simulink model "project"  (R2020b)
settings: Solver=VariableStepAuto  StartTime=0.0  StopTime=10  RelTol=1e-3
undefined symbols (not defined in the file or in its folder): sigbuilder_block
settings Model: Creator=99003759  LastModifiedBy=99003759

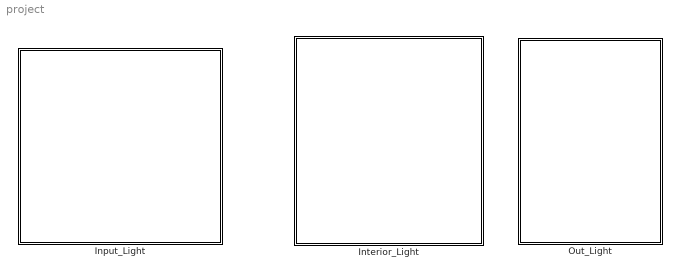
== system project ==
  Input_Light : Subsystem
  Interior_Light : Subsystem
  Out_Light : Subsystem

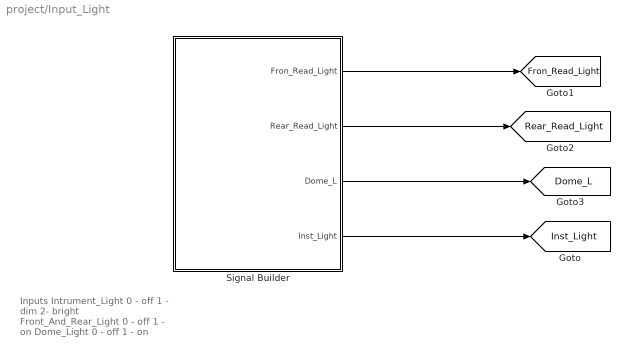
== system project/Input_Light ==
  note: Inputs
      | Intrument_Light
      | 0 - off
      | 1 - dim
      | 2- bright
      | Front_And_Rear_Light
      | 0 - off
      | 1 - on
      | Dome_Light
      | 0 - off
      | 1 - on
  Signal Builder : Subsystem  Tag=STV Subsys  LoadFcn=sigbuilder_block('load');  StartFcn=sigbuilder_block('start');  StopFcn=sigbuilder_block('stop');  ClipboardFcn=sigbuilder_block('clipboard');  mask(Sigbuilder block){tuvar=[0:10]}
      mask help: Simulink:masks:SigbuilderBlock_MD
      mask init:
      | if ~strcmp(get_param(bdroot(gcbh),'SimulationStatus'),'stopped') tuvar = sigbuilder_block('maskInit'); end
      settings: CopyFcn=sigbuilder_block('copy');  DeleteFcn=sigbuilder_block('delete');  ModelCloseFcn=sigbuilder_block('modelClose');  PreSaveFcn=sigbuilder_block('preSave');  PauseFcn=sigbuilder_block('pause');  ContinueFcn=sigbuilder_block('continue');  NameChangeFcn=sigbuilder_block('namechange');  OpenFcn=sigbuilder_block('open',[373.5 207 544.5 355.5 ]);  CloseFcn=sigbuilder_block('close');
      mask Display: plot(0, 0, 100, 100,[2, 2, 32, 32, 2], [68, 8, 8, 68, 68],[32, 2], [38, 38], [32, 19, 2],[53, 60, 44], [32, 17, 17, 2],[16, 16, 31, 31]);txt = getActiveGroup(gcbh);text(2, 100, txt,'verticalAlignment', 'top');
  tag scope: Dome_L=global, Fron_Read_Light=global, Inst_Light=global, Rear_Read_Light=global
  wires:
  Signal Builder/4(Inst_Light) -> [Inst_Light]
  Signal Builder/1(Fron_Read_Light) -> [Fron_Read_Light]
  Signal Builder/2(Rear_Read_Light) -> [Rear_Read_Light]
  Signal Builder/3(Dome_L) -> [Dome_L]

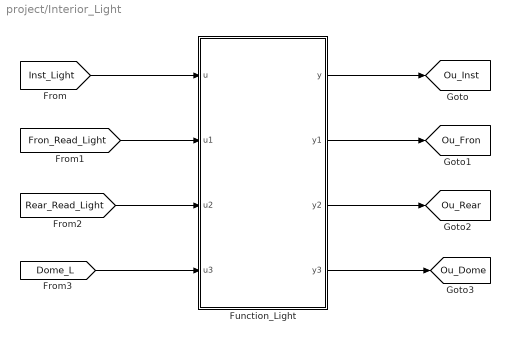
== system project/Interior_Light ==
  Function_Light : MATLAB Function  TreatAsAtomicUnit=on
  tag scope: Ou_Dome=global, Ou_Fron=global, Ou_Inst=global, Ou_Rear=global
  wires:
  [Dome_L] -> Function_Light/4(u3)
  [Inst_Light] -> Function_Light/1(u)
  [Fron_Read_Light] -> Function_Light/2(u1)
  [Rear_Read_Light] -> Function_Light/3(u2)
  Function_Light/1(y) -> [Ou_Inst]
  Function_Light/2(y1) -> [Ou_Fron]
  Function_Light/3(y2) -> [Ou_Rear]
  Function_Light/4(y3) -> [Ou_Dome]

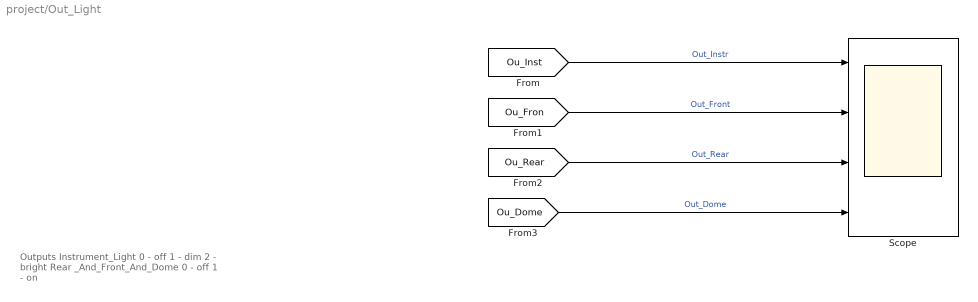
== system project/Out_Light ==
  note: Outputs
      | Instrument_Light
      | 0 - off
      | 1 - dim
      | 2 - bright
      | Rear _And_Front_And_Dome
      | 0 - off
      | 1 - on
  Scope : Scope  NumInputPorts=4
  wires:
  [Ou_Fron] -> Scope/2  "Out_Front"
  [Ou_Rear] -> Scope/3  "Out_Rear"
  [Ou_Dome] -> Scope/4  "Out_Dome"
  [Ou_Inst] -> Scope/1  "Out_Instr"

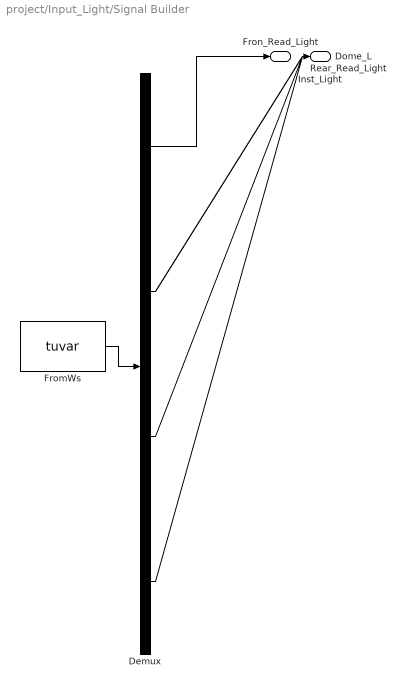
== system project/Input_Light/Signal Builder ==
  Demux : Demux  Tag=STV Demux
      settings: DisplayOption=none
  FromWs : FromWorkspace  Tag=STV FromWs  VariableName=tuvar
      SigBuilderData=|
      | common.afterFinalStr = 'Extrapolate'
      | common.sampleTime = 0
      | dataSet.timeRange = [0 10]
      | dataSet.name = 'Group 1'
      | sbobj.Groups.Name = 'Group 1'
      | sbobj.Groups.Signals(1).Name = 'Fron_Read_Light'
      | sbobj.Groups.Signals(1).XData = [0 0.5 0.5 1 1 1.5 1.5 2 2 2.5 2.5 3 3 3.5 3.5 4 4 4.5 4.5 5 5 5.5 5.5 6 6 6.5 6.5 7 7 7.5 7.5 8 8 8.5 8.5 9 9 9.5 9.5 10]
      | sbobj.Groups.Signals(1).YData = [2 2 0 0 2 2 0 0 2 2 0 0 2 2 0 0 2 2 0 0 2 2 0 0 2 2 0 0 2 2 0 0 2 2 0 0 2 2 0 0]
      | sbobj.Groups.Signals(2).Name = 'Rear_Read_Light'
      | sbobj.Groups.Signals(2).XData = [0 0.5 0.5 1 1 1.5 1.5 2 2 2.5 2.5 3 3 3.5 3.5 4 4 4.5 4.5 5 5 5.5 5.5 6 6 6.5 6.5 7 7 7.5 7.5 8 8 8.5 8.5 9 9 9.5 9.5 10]
      | sbobj.Groups.Signals(2).YData = [2 2 0 0 2 2 0 0 2 2 0 0 2 2 0 0 2 2 0 0 2 2 0 0 2 2 0 0 2 2 0 0 2 2 0 0 2 2 0 0]
      | sbobj.Groups.Signals(3).Name = 'Dome_L'
      | sbobj.Groups.Signals(3).XData = [0 0.5 0.5 1 1 1.5 1.5 2 2 2.5 2.5 3 3 3.5 3.5 4 4 4.5 4.5 5 5 5.5 5.5 6 6 6.5 6.5 7 7 7.5 7.5 8 8 8.5 8.5 9 9 9.5 9.5 10]
      | sbobj.Groups.Signals(3).YData = [2 2 0 0 2 2 0 0 2 2 0 0 2 2 0 0 2 2 0 0 2 2 0 0 2 2 0 0 2 2 0 0 2 2 0 0 2 2 0 0]
      | sbobj.Groups.Signals(4).Name = 'Inst_Light'
      | sbobj.Groups.Signals(4).XData = [0 1 2 3 4 5 6 7 8 9 10]
      | sbobj.Groups.Signals(4).YData = [0 0 1 2 0 2 1 0 1 2 0]
  Fron_Read_Light : Outport  Tag=STV Outport
  Rear_Read_Light : Outport  Tag=STV Outport  Port=2
  Dome_L : Outport  Tag=STV Outport  Port=3
  Inst_Light : Outport  Tag=STV Outport  Port=4
  wires:
  FromWs/1 -> Demux/1
  Demux/1 -> Fron_Read_Light/1
  Demux/2 -> Rear_Read_Light/1
  Demux/3 -> Dome_L/1
  Demux/4 -> Inst_Light/1

== matlab function project/Interior_Light/Function_Light ==
  data: u input; y output; u1 input; y1 output; u2 input; y2 output; u3 input; y3 output
function [y,y1,y2,y3] = fcn(u,u1,u2,u3)

y3 = u3;
y2 = u2;
y1 = u1;
y = u;
